simulink model "model4"  (R2024a)
settings: Solver=VariableStepAuto  StartTime=0.0  StopTime=10.0  RelTol=1e-3
values from neighbouring files (symbols this model uses):
  A = 1    [modelSave.m]    (also in s4.m = [5 -9 -7 1)
  B = 1    [modelSave.m]    (also in s4.m = [3; 3; 1; 3])
  C = 1    [modelSave.m]    (also in s4.m = [0 1 0 0)
  D = 1    [modelSave.m]    (also in s4.m = [4; 1])
  Gamma = 1    [modelSave.m]    (also in s4.m = diag([-10 -15]))
  K = 1    [modelSave.m]    (also in s4.m = place(A,B,[-3 -3+4i -3-4i -5]))
  Q = 1    [modelSave.m]    (also in s4.m = lyap(-Gamma, A, -Y*C))
  Y = 1    [modelSave.m]    (also in s4.m = [3 2; 1 4])
settings Model: Creator=eva  LastModifiedBy=eva

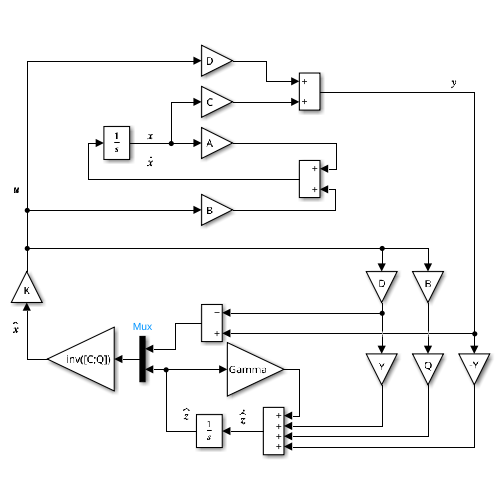
[thumbnail: Simulink's stored preview of the top-level diagram]
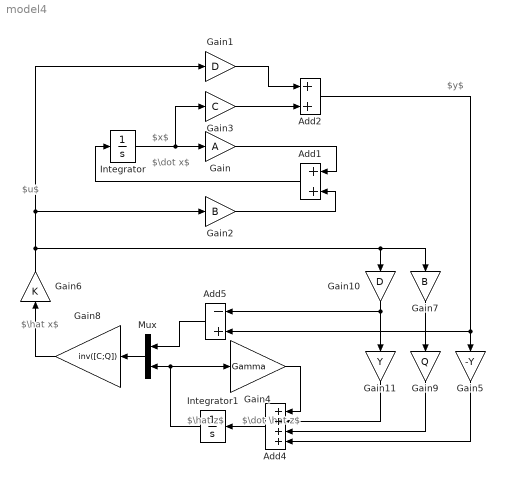
== system model4 ==
  note: $\dot \hat z$
  note: $y$
  note: $\dot x$
  note: $u$
  note: $x$
  note: $\hat z$
  note: $\hat x$
  Add1 : Sum
  Add2 : Sum
  Add4 : Sum  Inputs=++++
  Add5 : Sum  Inputs=-+
  Gain : Gain  Gain=A
  Gain1 : Gain  Gain=D
  Gain10 : Gain  Gain=D
  Gain11 : Gain  Gain=Y
  Gain2 : Gain  Gain=B
  Gain3 : Gain  Gain=C
  Gain4 : Gain  Gain=Gamma
  Gain5 : Gain  Gain=-Y
  Gain6 : Gain  Gain=K
  Gain7 : Gain  Gain=B
  Gain8 : Gain  Gain=inv([C;Q])
  Gain9 : Gain  Gain=Q
  Integrator : Integrator
  Integrator1 : Integrator
  Mux : Mux  Inputs=2
  wires:
  Integrator/1 -> Gain3/1, Gain/1
  Gain/1 -> Add1/1
  Gain2/1 -> Add1/2
  Add1/1 -> Integrator/1
  Gain3/1 -> Add2/2
  Gain1/1 -> Add2/1
  Add2/1 -> Gain5/1, Add5/2
  Gain7/1 -> Gain9/1
  Gain10/1 -> Add5/1, Gain11/1
  Gain11/1 -> Add4/2
  Add4/1 -> Integrator1/1
  Integrator1/1 -> Gain4/1, Mux/2
  Add5/1 -> Mux/1
  Gain6/1 -> Gain10/1, Gain7/1, Gain1/1, Gain2/1
  Mux/1 -> Gain8/1
  Gain8/1 -> Gain6/1
  Gain4/1 -> Add4/1
  Gain5/1 -> Add4/4
  Gain9/1 -> Add4/3
